simulink model "Simulink_WMM"  (R2021a)
settings: Solver=ode1be  StartTime=0.0  StopTime=350  FixedStep=0.001  RelTol=1e-3
values from neighbouring files (symbols this model uses):
  s = cross(t,r)    [traj_plan_circle.m]
  Y = 0    [traj_plan_3priority.m]    (also in traj_plan_double2.m; traj_plan_ee_8.m; traj_plan_ee_circle.m; traj_plan_scene.m)
undefined symbols (not defined in the file or in its folder): X, Z
libraries: sm_lib x132, nesl_utility x61
(part 4 of 4)

== matlab function Simulink_WMM/ /MATLAB Function2 ==
  data: x input; xyzrpy output; y input; z input; R input
function xyzrpy = xyzR2xyzrpy(x,y,z,R)


if abs(R(3 ,1) - 1.0) < 1.0e-15   % singularity
    a = 0.0;
    b = -pi / 2.0;
    c = atan2(-R(1, 2), -R(1, 3));
elseif abs(R(3, 1) + 1.0) < 1.0e-15   % singularity
    a = 0.0;
    b = pi / 2.0;
    c = -atan2(R(1, 2), R(1, 3));
else
    a = atan2(R(3, 2), R(3, 3));
    c = atan2(R(2, 1), R(1, 1));
    %     a = atan2(-R(3, 2), -R(3, 3));  %a另一个解
    %     c = atan2(-R(2, 1), -R(1, 1));  %c另一个解
    cosC = cos(c);
    sinC = sin(c);
    
    if abs(cosC) > abs(sinC)
        b = atan2(-R(3, 1), R(1, 1) / cosC);
    else
        b = atan2(-R(3, 1), R(2, 1) / sinC);
    end
end

rpy = [a, b, c];

xyzrpy = [x;y;z;rpy'];

== matlab function Simulink_WMM/Subsystem/MATLAB Function2 ==
  data: xyzrpy_d input; dxyzwxyz_d input; xyth_d input; dxyth_d input; q input; xyzrpy_WE input; dq_c output; xyzrpy_W0 input; xyzrpy_0E input
function dq_c= WMM_control(xyzrpy_d,dxyzwxyz_d,xyth_d,dxyth_d,q,xyzrpy_WE,xyzrpy_W0,xyzrpy_0E)
%% dq_c= WMM_controller(xyzrpy_d,dxyzwxyz_d,xyth_d,dxyth_d,q,xyzrpy_WE,xyzrpy_W0,xyzrpy_0E)
% 计算用于控制WMM的dq信号

% xyzrpy_d   ：规划的末端轨迹
% dxyzwxyz_d ：规划的末端速度
%  xyth_d    ：规划的车轨迹
%  dxyth_d   ：规划的车速度
%    q       ：实际运动的关节角
% xyzrpy_WE  ：世界系下臂末端的位姿
% xyzrpy_W0  ：世界系下车基座的位姿
% xyzrpy_0E  ：基座系下臂末端的位姿

%   dq_c     ：返回的关节速度控制信号

%%%%%%%%%%%%%%%%%%%%%%%%%%% 雅可比矩阵 %%%%%%%%%%%%%%%%%%%%%%%%%%%%%%%%%

    DH_table=build_DH_table_KinovaG3(q(3:end));
    Jm0=build_Jaco_manipulator(DH_table);
    R_W0=rotz(xyzrpy_W0(6)*180/pi);
    Jm=[R_W0,zeros(3,3);zeros(3,3),R_W0 ] * Jm0;
    Jb=build_Jaco_DWMR_base(xyzrpy_W0(6));
    Jaco1=[Jb,Jm];
    
%%%%%%%%%%%%%%%%%%%%% 第一优先级：控制末端dq_end %%%%%%%%%%%%%%%%%%%%%%

    K_ee=[28 30 20]'; % 末端控制P值
    dq_ee=pinv(Jaco1(1:3,:))*(dxyzwxyz_d(1:3)+K_ee.*(xyzrpy_d(1:3)-xyzrpy_WE(1:3)));

%%%%%%%%%%%%%%%%%%%%% 第二优先级：双轨迹dq_mobi %%%%%%%%%%%%%%%%%%%%%%%%%%%%

%     K_b=[0.1 0.1]'; % 车轨迹控制P值
%     Jaco_b=[Jb,0.*Jm];
%     N21=eye(size(Jaco1,2))-pinv(Jaco1(1:3,:))*Jaco1(1:3,:); % 投影矩阵：2投向1
%     Jaco2=Jaco_b*N21;
%     dxy_ee=Jaco_b*dq_ee;
%     Jaco2_pinv=Jaco_pinv(Jaco2(1:2,:));
%     dxy_c=dxyth_d(1:2)+K_b.*(xyth_d(1:2)-xyzrpy_W0(1:2));
%     dq_b=N21*Jaco2_pinv*(dxy_c-dxy_ee(1:2));

%%%%%%%%%%%%%% 第三优先级：避奇异避极限 dq_abnormal  dq_qlim %%%%%%%%%%%%%%%%

%     alpha_abnormal=100;
%     dq_abnormal_mani=alpha_abnormal.*grad_Hs(Jm);%机械臂避奇异
%     dq_abnormal=[0;0;dq_abnormal_mani];
% 
%     gamma=[1 1 1 1 1 1 1];
%     alpha_qlim=1;
%     dq_qlim_mani=-1.*alpha_qlim.*grad_Hl(Jm,q(3:end),gamma); % 避免关节限位
%     dq_qlim=[0;0;dq_qlim_mani];
%     
%     N32=eye(size(Jaco2,2))-Jaco2_pinv*Jaco2(1:2,:);  % 投影矩阵：3投向2
%     dq_3=N21*N32*(dq_abnormal + dq_qlim); 

%%%%%%%%%%%%%%%%%%%%%%%% 结果dq_c %%%%%%%%%%%%%%%%%%%%%%%%%%%

    dq_c = dq_ee ;%+ dq_b+ dq_3;
    
end

function grad_Hs = grad_Hs(Jaco)
% grad_Hs = grad_Hs(Jaco) 求奇异函数H(s)对qi的梯度
%   结果返回为 DoF 维列向量

n=size(Jaco,2);
grad_Hs=zeros(n,1);
    for i=1:n
        dJaco = Derivative_Jaco(Jaco);
        grad_Hs(i)=2.*det(Jaco*Jaco').*trace(dJaco(:,:,i)*pinv(Jaco));
    end
end

function grad_Hl = grad_Hl(Jaco,q,gamma)
% grad_Hl = grad_Hl(Jaco) 求奇异函数H(l)对qi的梯度
%   结果返回为 DoF 维列向量

n=size(Jaco,2);
qlim = build_qlim_KinovaG3; % 生成关节角度范围矩阵2×7，第一行为最小值
grad_Hl=zeros(n,1);
    for i=1:n
        grad_Hl(i)=1/gamma(i)...
                   .*(qlim(2,i)-qlim(1,i))^2 .* (2.*q(i)-qlim(2,i)-qlim(1,i))...
                   ./(q(i)-qlim(1,i))^2      ./ (qlim(2,i)-q(i))^2 ;
    end
end
